simulink library "m3_common_lib"  (R2021b)
settings: Solver=ode45  StartTime=0.0  StopTime=10.0  RelTol=1e-3
undefined symbols (not defined in the file or in its folder): ACCEL_PRE_MULT, APDT_SrvcMgr_IRVHVDCSubFcnReq, C_C1GearNumbers, C_C1GearRatios, C_Calibration, C_DitherWaveform, C_GearOffset, C_GearRatioIn, C_GearRatioInverseOut, C_GearRatioOut, CLUTCH_INNER_LOOP_UPDATE_RATE, CONSTANT, DEGRADED_MODE_SIZE, Dem_EventStatusType, DiscIntNeverNeededParam, F_FAULT_ENUM, F_NOFAULT, F_OUTOFRANGE, F_RATELIMIT, FALSE, FMI14_SPECIAL_INSTRUCTIONS, FMI20_DATA_DRIFTED_HIGH, FMI21_DATA_DRIFTED_LOW, FMI29_RESERVED_FOR_SAE_ASSIGNMENT, FMI30_RESERVED_FOR_SAE_ASSIGNMENT, FMI31_CONDITION_EXISTS, FMI32_NO_FAULT, IC, k_accel, k_mean, MAX_UINT32, MEAN_PRE_MULT, NTriggers, QLTY_SIGNAL_FAILED, QLTY_SIGNAL_FULLY_FUNCTION, QLTY_SIGNAL_SUBSTITUTED_BY_1ST_CHOICE, QLTY_SIGNAL_SUBSTITUTED_BY_2ND_CHOICE, QLTY_SIGNAL_SUBSTITUTED_BY_3RD_CHOICE, QLTY_SIGNAL_SUBSTITUTED_BY_4TH_CHOICE, SAMPLE_TIME_100us, simin, T_TestPoint, TF_FALSE, TF_TRUE, TimeStep, TRUE, WORKSPACE_UPDATE_RATE, Zero, ZERO
libraries: $bdroot x121, simulink x23, simulink_extras x4, MBD_EPS_Local_Blockset x4
(part 10 of 10)

== stateflow chart m3_common_lib/Diagnostics/DiagFaultCounter/DiagFaulCounter ==
  state FaultDebounceDisabled
    en: diagFaultStatus = Dem_EventStatusType.DEM_EVENT_STATUS_INIT;
    diagFaultCnt = int16(0);
    FaultDebounceDisabled -> (junction 32) [order 1]
    (junction 32) -> (junction 29) [order 1] : [~diagStartUpComp || diagReset || ~diagEnable]
        | {diagFaultStatus = Dem_EventStatusType.DEM_EVENT_STATUS_INIT;}
    (junction 32) -> (junction 23) [order 2]
    (junction 29) -> (junction 27)
    (junction 23) -> (junction 24) [order 1] : [~diagFaultActive]
        | {diagFaultStatus = Dem_EventStatusType.DEM_EVENT_STATUS_PREPASSED;}
    (junction 23) -> (junction 26) [order 2]
    (junction 24) -> (junction 282)
    (junction 26) -> (junction 281) [order 1] : [diagFaultActive]
        | {diagFaultStatus = Dem_EventStatusType.DEM_EVENT_STATUS_PREFAILED;}
    (junction 26) -> (junction 51) [order 2]
    (junction 281) -> (junction 283)
    (junction 283) -> (junction 51)
    (junction 282) -> (junction 283)
    (junction 27) -> (junction 282)
    (junction 51) -> (junction 288)
  state FaultDebounceEnabled
    en: diagFaultStatus = Dem_EventStatusType.DEM_EVENT_STATUS_INIT;
    diagFaultCnt = int16(0);
    state Init
      en: diagFaultCnt = int16(0);
      diagFaultStatus = Dem_EventStatusType.DEM_EVENT_STATUS_INIT;
      Init -> (junction 248) [order 1]
      (junction 248) -> (junction 249) [order 1] : [~diagStartUpComp || diagReset || ~diagEnable]
          | {diagFaultCnt = int16(0);}
      (junction 248) -> (junction 250) [order 2]
      (junction 249) -> (junction 257)
      (junction 250) -> (junction 253) [order 1] : [~diagFaultActive]
          | {diagFaultCnt = diagFaultCnt - diagDnCnt;}
      (junction 253) -> (junction 342) [order 1] : [diagFaultCnt<=diagPassCntThresh]
          | {diagFaultStatus = Dem_EventStatusType.DEM_EVENT_STATUS_PASSED;}
      (junction 250) -> (junction 252) [order 2]
      (junction 253) -> (junction 255) [order 2]
      (junction 342) -> (junction 344)
      (junction 252) -> (junction 251) [order 1] : [diagFaultActive]
          | {diagFaultCnt = diagFaultCnt + diagUpCnt;}
      (junction 251) -> (junction 310) [order 1] : [diagFaultCnt>=diagFaultCntThresh]
          | {diagFaultStatus = Dem_EventStatusType.DEM_EVENT_STATUS_FAILED;}
      (junction 251) -> (junction 256) [order 2]
      (junction 310) -> (junction 338)
      (junction 252) -> (junction 254) [order 2]
      (junction 256) -> (junction 254)
      (junction 338) -> (junction 256)
      (junction 255) -> (junction 338)
      (junction 344) -> (junction 255)
      (junction 257) -> (junction 344)
      (junction 254) -> (junction 258)
    state Fault
      en: diagFaultCnt = int16(0);
      diagFaultStatus = Dem_EventStatusType.DEM_EVENT_STATUS_FAILED;
      Fault -> (junction 133) [order 1]
      (junction 133) -> (junction 134) [order 1] : [(diagFaultCnt<int16(0)) && diagFaultActive]
          | {diagFaultCnt = diagFaultCnt + diagUpCnt;}
      (junction 134) -> (junction 152) [order 1] : [diagFaultCnt>int16(0)]
          | {diagFaultCnt = int16(0)}
      (junction 133) -> (junction 135) [order 2]
      (junction 134) -> (junction 139) [order 2]
      (junction 152) -> (junction 155)
      (junction 135) -> (junction 136) [order 1] : [~diagFaultActive && diagHealEn]
          | {diagFaultCnt = diagFaultCnt - diagDnCnt;}
      (junction 136) -> (junction 298) [order 1] : [diagFaultCnt<=diagPassCntThresh]
          | {diagFaultStatus = Dem_EventStatusType.DEM_EVENT_STATUS_PASSED;}
      (junction 135) -> (junction 137) [order 2]
      (junction 136) -> (junction 138) [order 2]
      (junction 298) -> (junction 300)
      (junction 138) -> (junction 137)
      (junction 300) -> (junction 138)
      (junction 139) -> (junction 300)
      (junction 155) -> (junction 139)
      (junction 137) -> (junction 140)
    state Pass
      en: diagFaultCnt = int16(0);
      diagFaultStatus = Dem_EventStatusType.DEM_EVENT_STATUS_PASSED;
      Pass -> (junction 159) [order 1]
      (junction 159) -> (junction 160) [order 1] : [(diagFaultCnt>int16(0)) && ~diagFaultActive]
          | {diagFaultCnt = diagFaultCnt - diagDnCnt;}
      (junction 160) -> (junction 161) [order 1] : [diagFaultCnt<int16(0)]
          | {diagFaultCnt = int16(0)}
      (junction 159) -> (junction 162) [order 2]
      (junction 160) -> (junction 166) [order 2]
      (junction 161) -> (junction 167)
      (junction 162) -> (junction 163) [order 1] : [diagFaultActive]
          | {diagFaultCnt = diagFaultCnt + diagUpCnt;}
      (junction 163) -> (junction 305) [order 1] : [diagFaultCnt>=diagFaultCntThresh]
          | {diagFaultStatus = Dem_EventStatusType.DEM_EVENT_STATUS_FAILED;}
      (junction 162) -> (junction 164) [order 2]
      (junction 163) -> (junction 165) [order 2]
      (junction 305) -> (junction 304)
      (junction 165) -> (junction 164)
      (junction 304) -> (junction 165)
      (junction 166) -> (junction 304)
      (junction 167) -> (junction 166)
      (junction 164) -> (junction 168)
    (default) -> Init
    Init -> Fault [order 1] : [diagFaultCnt>=diagFaultCntThresh &&...
        | diagStartUpComp &&...
        | ~diagReset && diagEnable]
    Fault -> Init [order 2] : [~diagStartUpComp ||...
        | diagReset || ~diagEnable]
    Fault -> Pass [order 1] : [diagFaultCnt<=diagPassCntThresh && diagHealEn]
    Pass -> Fault [order 1] : [diagFaultCnt>=diagFaultCntThresh]
    Init -> Pass [order 2] : [diagFaultCnt<=diagPassCntThresh &&...
        | diagStartUpComp &&...
        | ~diagReset && diagEnable]
    Pass -> Init [order 2] : [~diagStartUpComp ||...
        | diagReset || ~diagEnable]
  (default) -> (junction 58)
  (junction 58) -> (junction 279) [order 2]
  (junction 58) -> FaultDebounceEnabled [order 1] : [diagDbncEnab]
  (junction 279) -> FaultDebounceDisabled
  FaultDebounceEnabled -> FaultDebounceDisabled : [~diagDbncEnab]
  FaultDebounceDisabled -> FaultDebounceEnabled [order 1] : [diagDbncEnab]
  data: diagFaultActive input boolean size=1; diagStartUpComp input boolean size=1; diagReset input boolean size=1; diagEnable input boolean size=1; diagDbncEnab input boolean size=1; diagFaultCntThresh input int16 size=1; diagPassCntThresh input int16 size=1; diagUpCnt input int16 size=1; diagDnCnt input int16 size=1; diagFaultStatus output size=1; diagHealEn input boolean size=1; diagFaultCnt local int16 size=1
